simulink model "realTimeBatteryOPC"  (R2024a)
settings: Solver=FixedStepAuto  StartTime=0.0  StopTime=150000  RelTol=1e-3
values from neighbouring files (symbols this model uses):
  A = 0.00110214    [ConfiguracaoInicial.m]
  B = 0.000233175'    [ConfiguracaoInicial.m]
  C = 7.6408e-8    (= 7.6408e-08)    [ConfiguracaoInicial.m]
  cutoffVoltage = 3.65    [ConfiguracaoInicial.m]
  dischargeCutoffVoltage = 1.8    [ConfiguracaoInicial.m]
  finalPulse = 14    [ConfiguracaoInicial.m]
  hppcPulses = [0.05,0.05,0.05,0.05,0.1,0.1,0.1,0.1,0.1,0.1,0.05,0.05,0.05,0.05]    [ConfiguracaoInicial.m]
  initialCapacity = 1.45383    [ConfiguracaoInicial.m]
  initialSOC = 1.0    (= 1)    [ConfiguracaoInicial.m]
  initialState = 11    [ConfiguracaoInicial.m]
  loadCurrent = 1.45383    [ConfiguracaoInicial.m]
  maxCurrent = 100000000000000    [ConfiguracaoInicial.m]
  maxSOC = 10000000000.5    [ConfiguracaoInicial.m]
  maxTemperature = 800000000    [ConfiguracaoInicial.m]
  maxVoltage = 10000000.0    (= 10000000)    [ConfiguracaoInicial.m]
  minCurrent = -1000000000000    [ConfiguracaoInicial.m]
  minSOC = -10000000000.5    [ConfiguracaoInicial.m]
  minTemperature = -1500000    [ConfiguracaoInicial.m]
  minVoltage = -100000    [ConfiguracaoInicial.m]
  restChargeTimeHPPC = 3600*3    (= 10800)    [ConfiguracaoInicial.m]
  restTimeHPPC = 3600*2    (= 7200)    [ConfiguracaoInicial.m]
  Rt = 10000    [ConfiguracaoInicial.m]
  sampleTime = 0.01    [ConfiguracaoInicial.m]
  startDelay = 100    [ConfiguracaoInicial.m]
  startPulse = 1    [ConfiguracaoInicial.m]
undefined symbols (not defined in the file or in its folder): National_Instruments, PCIe, Standard_Devices, TCP_Protocol
libraries: eeGeneralControl x6, sldrtlib x5, slpidlib x1
settings Model: SimulationMode=external  ExtModeTrigDuration=180000  ExtModeArchiveMode=auto  ExtModeArchiveFileName=TesteComunicacao  ExtModeArchiveDirName=C:\Users\proje\OneDrive\Área de Trabalho\RealTimeBattery\Resultados Comunicacao  ExtModeWriteAllDataToWs=on  Creator=User  LastModifiedBy=proje
settings SolverCC: AlgebraicLoopSolver=TrustRegion  AutoInsertRateTranBlk=on  DecoupledContinuousIntegration=on  MinimalZcImpactIntegration=on
settings DataIOCC: ReturnWorkspaceOutputs=off
settings DebuggingCC: UnconnectedInputMsg=warning  UnconnectedOutputMsg=warning  UnconnectedLineMsg=warning  ArithmeticOperatorsInVariantConditions=warning
settings HardwareCC: ProdBitPerLong=64  ProdHWDeviceType=Intel->x86-64 (Linux 64)
settings ModelReferenceCC: EnableRefExpFcnMdlSchedulingChecks=on
settings SFSimCC: SimUseLocalCustomCode=off  CustomCodeUndefinedFunction=UseInterfaceOnly
settings RTWCC: Description=Simulink Desktop Real-Time  SystemTargetFile=sldrt.tlc  TemplateMakefile=sldrt.tmf  RTWUseLocalCustomCode=off  RTWCompilerOptimization=on  GPUComputeCapability=3.5  DLArmComputeVersion=19.05
settings CodeAppCC: MaxIdLength=95
settings SimulinkDesktopRealTimeCC: TargetLibSuffix=_sldrt.a  TargetPreCompLibLocation=C:\Program Files\MATLAB\R2024a\toolbox\sldrt\lib\win64
settings ConfigsetCC: ListOpcUaClients=[]  EndPoints=[]

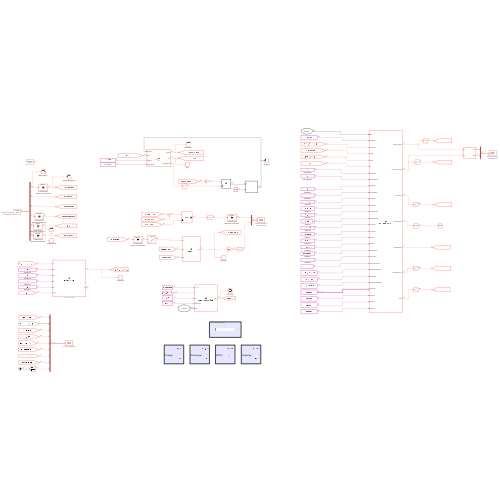
[thumbnail: Simulink's stored preview of the top-level diagram]
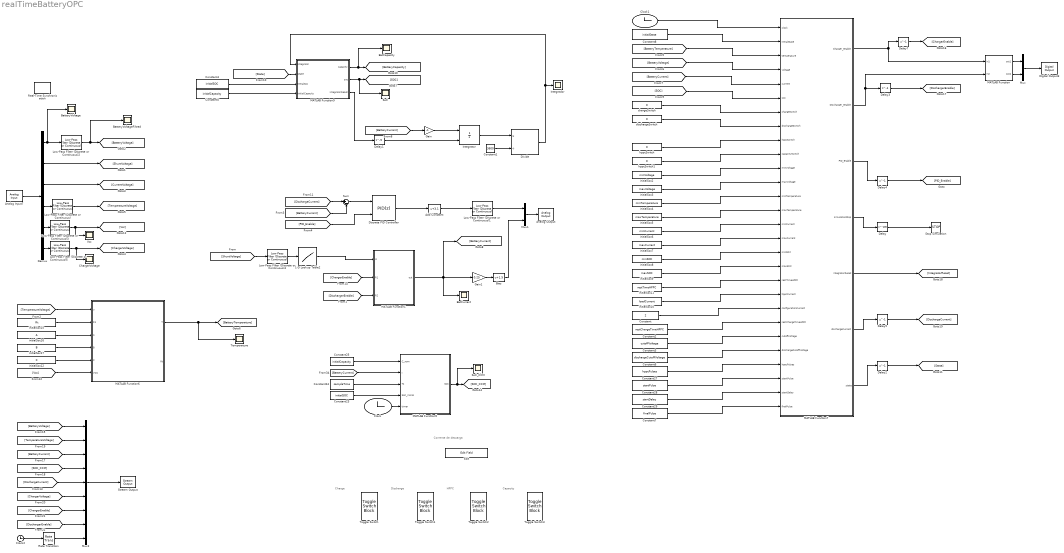
== system realTimeBatteryOPC ==
  note: Corrente de descarga
  note: Charge
  note: Discharge
  note: HPPC
  note: Capacity
  1-D Lookup Table2 : Lookup_n-D  NumberOfTableDimensions=1  BreakpointsForDimension1=|  Table=|  InternalRulePriority=Speed  RndMeth=Simplest
      BreakpointsForDimension1=|
      | [-0.703368941137097
      | -0.562690330092723
      | -0.492566163770883
      | -0.422967022263301
      | -0.352467845069619
      | -0.282288882664180
      | -0.247102233547827
      | -0.211796157294334
      | -0.176436693515434
      | -0.141402369117175
      | -0.106070485459359
      | -0.070887043775281
      | -0.035430249481695
      | -0.000072010558515
      | 0.035179496254845
      | 0.070319440336417
      | 0.105617401894233
      | 0.141115276831389
      | 0.176018947968660
      | 0.211326591943553
      | 0.246422461552550
      | 0.281747789595088
      | 0.351752022865883
      | 0.421762375644377
      | 0.491793233279879
      | 0.561360569786677
      | 0.701503863747804
      | ]
      Table=|
      | [-5.0040
      | -3.9980
      | -3.4995
      | -3.0010
      | -2.4995
      | -2.0000
      | -1.7500
      | -1.4990
      | -1.2490
      | -1.0005
      | -0.7495
      | -0.4995
      | -0.2490
      | 0.0000
      | 0.2500
      | 0.5000
      | 0.7500
      | 1.0020
      | 1.2505
      | 1.5005
      | 1.7505
      | 2.0020
      | 2.5000
      | 3.0000
      | 3.5005
      | 3.9985
      | 5.0025]
  Add Constant : Bias  Bias=3.1  SaturateOnIntegerOverflow=off
  Analog Input7 : sldrtlib/Analog Input  SampleTime=sampleTime  MaxMissedTicks=missedTicks  ShowMissedTicks=off  YieldWhenWaiting=off  DrvName=National_Instruments/PCIe-6323  DrvAddress=4294967295  DrvOptions=[1 127 63 0 0 0 0]  Channels=[1,2,3,4,5,6]  RangeMode=1  VoltRange=1  DataType=1
      settings: AttributesFormatString=National Instruments\nPCIe-6323 [auto]
  Analog Output : sldrtlib/Analog Output  SampleTime=sampleTime  MaxMissedTicks=missedTicks  ShowMissedTicks=off  YieldWhenWaiting=off  DrvName=National_Instruments/PCIe-6323  DrvAddress=4294967295  DrvOptions=[1 127 63 0 0 0 0]  Channels=[1,2]  RangeMode=1  VoltRange=1  InitialValue=0  FinalValue=0
      settings: AttributesFormatString=National Instruments\nPCIe-6323 [auto]
  BatCapacity : Scope
  BatCurrent : Scope
  BatteryVoltage : Scope
  BatteryVoltageFiltred : Scope
  Bias : Bias  Bias=1.5  SaturateOnIntegerOverflow=off
  ChargerVoltage : Scope
  Clock : Clock
  Clock1 : Clock
  Clock2 : Clock
  Constant : Constant  Value=2
  Constant1 : Constant  Value=3600
  Constant2 : Constant  Value=restChargeTimeHPPC
  Constant23 : Constant  Value=initialSOC
  Constant24 : Constant  Value=sampleTime
  Constant25 : Constant  Value=initialCapacity
  Constant27 : Constant  Value=hppcPulses
  Constant28 : Constant  Value=startPulse
  Constant29 : Constant  Value=startDelay
  Constant3 : Constant  Value=cutoffVoltage
  Constant4 : Constant  Value=initialSOC
  Constant5 : Constant  Value=initialCapacity
  Constant6 : Constant  Value=dischargeCutoffVoltage
  Constant7 : Constant  Value=finalPulse
  Constant8 : Constant  Value=initialState
  Delay : Delay  DelayLength=100  InitialCondition=0  SampleTime=sampleTime
  Delay1 : Delay  DelayLength=5  InitialCondition=0  SampleTime=sampleTime
  Delay2 : Delay  DelayLength=1  InitialCondition=0  SampleTime=sampleTime
  Delay{3..5,7} (4 alike) : Delay  DelayLength=1  InitialCondition=1  SampleTime=sampleTime
  Demux : Demux  Outputs=6
  Digital Output3 : sldrtlib/Digital Output  SampleTime=sampleTime  MaxMissedTicks=missedTicks  ShowMissedTicks=off  YieldWhenWaiting=off  DrvName=National_Instruments/PCIe-6323  DrvAddress=4294967295  DrvOptions=[1 127 63 0 0 0 0]  Channels=[2,1]  BitMode=1  InitialValue=[]  FinalValue=[]
      settings: AttributesFormatString=National Instruments\nPCIe-6323 [auto]
  Discrete PID Controller : slpidlib/PID Controller  Controller=PID  Form=Ideal  TimeDomain=Discrete-time  UseExternalTs=off  SampleTime=sampleTime  IntegratorMethod=Forward Euler  FilterMethod=Forward Euler  ControllerParametersSource=internal  P=0.07  I=0.007  UseKiTs=on  D=0.7  UseExternalDerivativeSource=off  N=10  UseFilter=on  TunerSelectOption=Transfer Function Based (PID Tuner App)  ZeroCross=off  InitialConditionSource=internal  InitialConditionForIntegrator=0  InitialConditionForFilter=0  DifferentiatorICPrevScaledInput=0  ExternalReset=level  TrackingMode=off  Kt=1  LimitOutput=on  SatLimitsSource=internal  UpperSaturationLimit=7  LowerSaturationLimit=0  LinearizeAsGain=off  AntiWindupMode=clamping  Kb=1  LimitIntegrator=off  UpperIntegratorSaturationLimit=5  LowerIntegratorSaturationLimit=-5  POutMin=[]  POutMax=[]  IOutMin=[]  IOutMax=[]  DOutMin=[]  DOutMax=[]  NOutMin=[]  NOutMax=[]  SumOutMin=[]  SumOutMax=[]  SaturationOutMin=[]  SaturationOutMax=[]  PParamMin=[]  PParamMax=[]  IParamMin=[]  IParamMax=[]  DParamMin=[]  DParamMax=[]  NParamMin=[]  NParamMax=[]  KbParamMin=[]  KbParamMax=[]  KtParamMin=[]  KtParamMax=[]  KbOutMin=[]  KbOutMax=[]  KtOutMin=[]  KtOutMax=[]  IntegratorOutMin=[]  IntegratorOutMax=[]  FilterOutMin=[]  FilterOutMax=[]  SumI1OutMin=[]  SumI1OutMax=[]  SumI2OutMin=[]  SumI2OutMax=[]  SumI3OutMin=[]  SumI3OutMax=[]  SumI4OutMin=[]  SumI4OutMax=[]  SumDOutMin=[]  SumDOutMax=[]  DifferentiatorOutMin=[]  DifferentiatorOutMax=[]  FilterDiffOutCoefMin=[]  FilterDiffOutCoefMax=[]  ReciprocalOutMin=[]  ReciprocalOutMax=[]  SumDenOutMin=[]  SumDenOutMax=[]  SumNumOutMin=[]  SumNumOutMax=[]  DivideOutMin=[]  DivideOutMax=[]  UdiffTsProdOutMin=[]  UdiffTsProdOutMax=[]  NTsProdOutMin=[]  NTsProdOutMax=[]  UintegralTsProdOutMin=[]  UintegralTsProdOutMax=[]  UngainTsProdOutMin=[]  UngainTsProdOutMax=[]  ClampingZeroOutDataTypeStr=Inherit: Inherit via back propagation  ClampingZeroOutMin=[]  ClampingZeroOutMax=[]  FilterDenConstantOutDataTypeStr=Inherit: Inherit via back propagation  FilterDenConstantOutMin=[]  FilterDenConstantOutMax=[]  PCopyOutDataTypeStr=Inherit: Inherit via back propagation  PCopyOutMin=[]  PCopyOutMax=[]  NCopyOutDataTypeStr=Inherit: Inherit via back propagation  NCopyOutMin=[]  NCopyOutMax=[]  IntegratorContinuousStateAttributes=''  IntegratorStateMustResolveToSignalObject=off  IntegratorRTWStateStorageClass=Auto  FilterContinuousStateAttributes=''  FilterStateMustResolveToSignalObject=off  FilterRTWStateStorageClass=Auto  ParallelPVariant=Passthrough  IdealPVariant=InternalParameters  IVariant=InternalParameters  DVariant=InternalParameters  IntegratorVariant=Discrete  SatVariant=Enabled  AWVariant=DiscClampingIdeal  PCopyVariant=InternalParamsIdeal  TRVariant=Disabled  FdbkBlocksVariant=Forward  IdealPFdbkVariant=Disabled  SatFdbkVariant=Disabled  DerivativeFilterVariant=ForwardEulerFilter  NVariant=InternalParameters  NCopyVariant=Disabled  FilterICVariant=InternalICsFilter  IntegratorICVariant=InternalICs  ExternalResetVariant=ExternalReset  TRSumVariant=Passthrough  SumFdbkVariant=Disabled  SumVariant=Sum_PID  TsampFilterVariant=InternalTs  TsampNgainVariant=Passthrough  TsampIntegralVariant=Disabled_SignalSpec  ExternalSaturationOutDataTypeStr=Inherit: Same as second input  DerivativeSourceVariant=ErrorSignal
      settings: LibrarySourceBlock=simulink/Discrete/Discrete PID Controller
  Divide : Product  Inputs=*/
  Edit : EditField  LabelPosition=Hide  ShowInitialText=on  Alignment=Center
  Gain : Gain  Gain=-1
  Gain1 : Gain  Gain=0.25
  Integrador : Scope
  Integrator : Integrator  ExternalReset=rising
  Low-Pass Filter (Discrete or Continuous) : eeGeneralControl/Low-Pass Filter (Discrete or Continuous)  K=1  T=1  B=inf  A=-inf  init_option=Specify as parameter  x0=2.5  Ts=sampleTime
  Low-Pass Filter (Discrete or Continuous)1 : eeGeneralControl/Low-Pass Filter (Discrete or Continuous)  K=1  T=1  B=inf  A=-inf  init_option=Specify as parameter  x0=0  Ts=sampleTime
  Low-Pass Filter (Discrete or Continuous)2 : eeGeneralControl/Low-Pass Filter (Discrete or Continuous)  K=1  T=1  B=inf  A=-inf  init_option=Specify as parameter  x0=0  Ts=sampleTime
  Low-Pass Filter (Discrete or Continuous)3 : eeGeneralControl/Low-Pass Filter (Discrete or Continuous)  K=1  T=1  B=inf  A=-inf  init_option=Specify as parameter  x0=5  Ts=sampleTime
  Low-Pass Filter (Discrete or Continuous)4 : eeGeneralControl/Low-Pass Filter (Discrete or Continuous)  K=1  T=1  B=inf  A=-inf  init_option=Specify as parameter  x0=0  Ts=sampleTime
  Low-Pass Filter (Discrete or Continuous)5 : eeGeneralControl/Low-Pass Filter (Discrete or Continuous)  K=1  T=1  B=inf  A=-inf  init_option=Specify as parameter  x0=3  Ts=sampleTime
  MATLAB Function : MATLAB Function  TreatAsAtomicUnit=on  SystemSampleTime=sampleTime
  MATLAB Function1 : MATLAB Function  TreatAsAtomicUnit=on  SystemSampleTime=sampleTime
  MATLAB Function5 : MATLAB Function  TreatAsAtomicUnit=on  SystemSampleTime=sampleTime
  MATLAB Function6 : MATLAB Function  TreatAsAtomicUnit=on  SystemSampleTime=sampleTime
  MATLAB Function7 : MATLAB Function  TreatAsAtomicUnit=on  SystemSampleTime=sampleTime
  MATLAB Function9 : MATLAB Function  TreatAsAtomicUnit=on  SystemSampleTime=sampleTime
  Mux : Mux  Inputs=2
  Mux1 : Mux  Inputs=2
  Mux2 : Mux  Inputs=9
  Rate Transition : RateTransition  OutPortSampleTime=sampleTime
  Real-Time Synchronization : sldrtlib/Real-Time Synchronization  SampleTime=sampleTime  MaxMissedTicks=missedTicks  ShowMissedTicks=on  YieldWhenWaiting=off
  SoC : Scope
  SoC_CCM : Scope
  Stop Simulation : Stop
  Stream Output : sldrtlib/Stream Output  SampleTime=sampleTime  MaxMissedTicks=10  ShowMissedTicks=off  YieldWhenWaiting=off  DrvName=Standard_Devices/TCP_Protocol  DrvAddress=16384  DrvOptions=[0 8081 49 57 50 46 49 54 56 46 48 46 50 51 49 0 0 0 0 0 0 0 0 0 0 0 0 0 0 0 0 0 0 0 0 0 0 0 0 0 0 0 0 0 0 0 0 0 0 0 0 0 0 0 0 0 0 0 0 0 0 0 0 0 0 0 0 0 0 0 0 0 0 0 0 0 0 0 0 0 0 0 0 0 0 0 0 0 0 0 0 0 0 0 0 0 0 0 0 0 0 0 0 0 0 0 0 0 0 0 0 0 0 0 0 0 0 0 0 0 0 0 0 0 0 0 0 0 0 0 0 0 0 0 0 0 0 0 0 0 0 0 0 0 0 0 0 0 0 0 0 0 0 0 0 0 0 0 0 0 0 0 0 0 0 0 0 0 0 0 0 0 0 0 0 0 0 0 0 0 0 0 0 0 0 0 0 0 0 0 0 0 0 0 0 0 0 0 0 0 0 0 0 0 0 0 0 0 0 0 0 0 0 0 0 0 0 0 0 0 0 0 0 0 0 0 0 0 0 0 0 0 0 0 0 0 0 0 0 0 0 0 0 0 0 0 0 0 0 0 0 0 0 0 0 0]  PortSizes=9  FormatString="\"<%lf:%lf:%lf:%lf:%lf:%lf:%lf:%lf:%lf>\""  ShowReady=off  ShowError=off  InitialValue=[]  FinalValue=[]
      settings: AttributesFormatString=TCP Protocol [16384]
  Sum : Sum  Inputs=|+-
  Temperature : Scope
  Toggle Switch{,1..3} (4 alike) : ToggleSwitchBlock
      settings: Values={{'Off', 'On'}, [0 1]}
  Vcc : Scope
  chargeSwitch : Constant  Value=0
  dischargeSwitch : Constant  Value=0
  hppcSwitch : Constant  Value=0
  hppcSwitch1 : Constant  Value=0
  initialSoc10 : Constant  Value=loadCurrent
  initialSoc11 : Constant  Value=restTimeHPPC
  initialSoc12 : Constant  Value=C
  initialSoc15 : Constant  Value=Rt
  initialSoc16 : Constant  Value=A
  initialSoc17 : Constant  Value=B
  initialSoc2 : Constant  Value=minVoltage
  initialSoc3 : Constant  Value=maxVoltage
  initialSoc4 : Constant  Value=minTemperature
  initialSoc5 : Constant  Value=maxTemperature
  initialSoc6 : Constant  Value=minCurrent
  initialSoc7 : Constant  Value=maxCurrent
  initialSoc8 : Constant  Value=minSOC
  initialSoc9 : Constant  Value=maxSOC
  wires:
  Clock1/1 -> MATLAB Function7/1(clock)
  MATLAB Function7/1(Charger_Enable) -> Delay7/1, MATLAB Function/1(in1)
  Demux/1 -> Low-Pass Filter (Discrete or Continuous)2/1, BatteryVoltage/1
  [BatteryTemperature] -> MATLAB Function7/3(temperature)
  [BatteryVoltage] -> MATLAB Function7/4(voltage)
  [BatteryCurrent] -> MATLAB Function7/5(current)
  Gain/1 -> Integrator/1
  [BatteryCurrent] -> Gain/1
  [SOC] -> MATLAB Function7/6(soc)
  MATLAB Function7/4(simulationStop) -> Delay/1
  Delay/1 -> Stop Simulation/1
  initialSoc4/1 -> MATLAB Function7/13(minTemperature)
  initialSoc3/1 -> MATLAB Function7/12(maxVoltage)
  initialSoc2/1 -> MATLAB Function7/11(minVoltage)
  initialSoc5/1 -> MATLAB Function7/14(maxTemperature)
  initialSoc6/1 -> MATLAB Function7/15(minCurrent)
  initialSoc7/1 -> MATLAB Function7/16(maxCurrent)
  initialSoc8/1 -> MATLAB Function7/17(minSOC)
  initialSoc9/1 -> MATLAB Function7/18(maxSOC)
  initialSoc11/1 -> MATLAB Function7/19(restTimeHPPC)
  initialSoc15/1 -> MATLAB Function6/2(R1)
  chargeSwitch/1 -> MATLAB Function7/7(chargeSwitch)
  dischargeSwitch/1 -> MATLAB Function7/8(dischargeSwitch)
  hppcSwitch/1 -> MATLAB Function7/9(hppcSwitch)
  [BatteryCurrent] -> Sum/2
  Sum/1 -> Discrete PID Controller/1
  Integrator/1 -> Divide/1
  Constant1/1 -> Divide/2
  initialSoc10/1 -> MATLAB Function7/20(hppcCurrent)
  MATLAB Function7/5(integratorReset) -> [IntegratorReset]
  MATLAB Function7/6(dischargeCurrent) -> Delay5/1
  [DischargeCurrent] -> Sum/1
  MATLAB Function9/1(capacity) -> BatCapacity/1, [BatteryCapacity]
  MATLAB Function9/2(soc) -> SoC/1, [SOC]
  Delay1/1 -> Integrator/2
  [State] -> MATLAB Function9/2(state)
  [TemperatureVoltage] -> MATLAB Function6/1(u)
  initialSoc12/1 -> MATLAB Function6/5(C)
  initialSoc17/1 -> MATLAB Function6/4(B)
  initialSoc16/1 -> MATLAB Function6/3(A)
  Constant/1 -> MATLAB Function7/21(configurationCurrent)
  Constant2/1 -> MATLAB Function7/22(restChargeTimeHPPC)
  Delay3/1 -> [DischargerEnable]
  MATLAB Function7/2(Discharger_Enable) -> MATLAB Function/2(in2), Delay3/1
  MATLAB Function7/3(PID_Enable) -> Delay4/1
  Delay4/1 -> [PID_Enable]
  Delay5/1 -> [DischargeCurrent]
  MATLAB Function7/7(state) -> Delay2/1
  MATLAB Function9/3(integratorReset) -> Delay1/1
  Constant3/1 -> MATLAB Function7/23(cutoffVoltage)
  Constant4/1 -> MATLAB Function9/3(initialSoc)
  Constant5/1 -> MATLAB Function9/4(initialCapacity)
  Delay2/1 -> [State]
  Divide/1 -> MATLAB Function9/1(integrator), Integrador/1
  Constant8/1 -> MATLAB Function7/2(initialState)
  [Vcc] -> MATLAB Function6/6(VCC)
  hppcSwitch1/1 -> MATLAB Function7/10(capacitySwitch)
  [ShuntVoltage] -> Low-Pass Filter (Discrete or Continuous)4/1
  Low-Pass Filter (Discrete or Continuous)4/1 -> 1-D Lookup Table2/1
  Gain1/1 -> Bias/1
  Constant24/1 -> MATLAB Function5/3(Ts)
  [BatteryCurrent] -> MATLAB Function5/2(I)
  MATLAB Function5/1(SoC) -> SoC_CCM/1, [SOC_CCM]
  Constant25/1 -> MATLAB Function5/1(C_nom)
  Clock/1 -> MATLAB Function5/5(timer)
  Analog Input7/1 -> Demux/1
  Mux/1 -> Digital Output3/1
  Constant27/1 -> MATLAB Function7/25(hppcPulses)
  Constant28/1 -> MATLAB Function7/26(startPulse)
  Constant29/1 -> MATLAB Function7/27(startDelay)
  Constant23/1 -> MATLAB Function5/4(SoC_Inicial)
  Bias/1 -> Mux1/2
  Mux1/1 -> Analog Output/1
  Demux/6 -> Low-Pass Filter (Discrete or Continuous)5/1
  Demux/5 -> Low-Pass Filter (Discrete or Continuous)3/1
  Demux/4 -> Low-Pass Filter (Discrete or Continuous)/1
  Demux/2 -> [ShuntVoltage]
  Demux/3 -> [CurrentVoltage]
  [PID_Enable] -> Discrete PID Controller/2
  Discrete PID Controller/1 -> Add Constant/1
  Add Constant/1 -> Low-Pass Filter (Discrete or Continuous)1/1
  Low-Pass Filter (Discrete or Continuous)1/1 -> Mux1/1
  Constant6/1 -> MATLAB Function7/24(dischargeCutoffVoltage)
  Constant7/1 -> MATLAB Function7/28(finalPulse)
  1-D Lookup Table2/1 -> MATLAB Function1/1(in)
  [ChargerEnable] -> MATLAB Function1/2(R1)
  [DischargerEnable] -> MATLAB Function1/3(R2)
  MATLAB Function1/1(out) -> [BatteryCurrent], BatCurrent/1, Gain1/1
  Low-Pass Filter (Discrete or Continuous)2/1 -> BatteryVoltageFiltred/1, [BatteryVoltage]
  Delay7/1 -> [ChargerEnable]
  [BatteryVoltage] -> Mux2/1
  Mux2/1 -> Stream Output/1
  [TemperatureVoltage] -> Mux2/2
  [BatteryCurrent] -> Mux2/3
  [SOC_CCM] -> Mux2/4
  [ChargerVoltage] -> Mux2/6
  [ChargerEnable] -> Mux2/7
  [DischargerEnable] -> Mux2/8
  Clock2/1 -> Rate Transition/1
  Rate Transition/1 -> Mux2/9
  [DischargeCurrent] -> Mux2/5
  MATLAB Function/2(out2) -> Mux/2
  MATLAB Function/1(out1) -> Mux/1
  MATLAB Function6/1(T) -> Temperature/1, [BatteryTemperature]
  Low-Pass Filter (Discrete or Continuous)/1 -> [TemperatureVoltage]
  Low-Pass Filter (Discrete or Continuous)3/1 -> Vcc/1, [Vcc]
  Low-Pass Filter (Discrete or Continuous)5/1 -> ChargerVoltage/1, [ChargerVoltage]

== matlab function realTimeBatteryOPC/MATLAB Function9 ==
  data: integrator input; state input; capacity output; soc output; integratorReset output; initialSoc input; initialCapacity input
function [capacity, soc, integratorReset] = calculate_capacity(integrator, state, initialSoc,initialCapacity)
    persistent current_capacity; % Definindo a capacidade como persistente
    persistent socRef;
    persistent previousState;
    
    if isempty(current_capacity) % Verificando se a capacidade atual está vazia
        current_capacity = initialCapacity; % Definindo a capacidade inicial como zero
        socRef=initialSoc;
        previousState=0;
    end
    integratorReset=0;

    if state==1 && previousState==0
        socRef=0;
        integratorReset=1;
    elseif state==4 && previousState==3 && abs(integrator)> current_capacity
        current_capacity = abs(integrator); 
        integratorReset=1;
        socRef=1;
    elseif state==5 && previousState==4
        integratorReset=1;
        socRef=1;
    elseif state==6 && previousState==5 && abs(integrator)>current_capacity
        current_capacity = abs(integrator); 
        integratorReset=1;
        socRef=0;
    elseif state==7 && previousState==6
        integratorReset=1;
        socRef=0;
    elseif state==10 && previousState==9 && abs(integrator)>current_capacity
        %current_capacity = abs(integrator); 
        integratorReset=1;
        socRef=1;
    elseif state==11 && previousState==1-0 
        integratorReset=1;
        socRef=1;
    end
    
    previousState=state;

    capacity = current_capacity; % Retornando a capacidade atual

    soc=socRef+integrator/current_capacity;

    if(soc<-0.1) 
        soc=-0.1;
    end

    if(soc>1.1) 
        soc=1.1;
    end
end

== matlab function realTimeBatteryOPC/MATLAB Function1 ==
  data: in input; R1 input; R2 input; out output
function out  = currentOn(in, R1, R2) 

    if(R1==1 || R2==1)
        out=in;
    else
        out=0;
    end

end

== matlab function realTimeBatteryOPC/MATLAB Function ==
  data: in1 input; out1 output; in2 input; out2 output
function [out1, out2] = fcn(in1, in2)
    % Definir variáveis persistentes para armazenar o estado anterior
    persistent previousIn2;
    
    % Inicializar as variáveis persistentes na primeira execução
    if isempty(previousIn2)
        previousIn2 = 0;
    end

    if(previousIn2==0 && in2==1)
        out1=0;
        out2=1;
    elseif(previousIn2==1 && in2==0)
        out1=0;
        out2=1;
    elseif(in2==1)
        out2=1;
        out1=1;
    else
        out2=0;
        out1=in1;
    end

    
    previousIn2=in2;

end

== matlab function realTimeBatteryOPC/MATLAB Function5 ==
  data: C_nom input; SoC output; I input; Ts input; SoC_Inicial input; timer input
function SoC = coulomb_counting_SOC(C_nom, I, Ts, SoC_Inicial,timer)
% Este código implementa a contagem de Coulomb usando um integrador discreto
% com o método do trapézio, utilizando variáveis persistentes.
% C_nom: Capacidade nominal da bateria (Ah)
% I: Corrente da bateria (A)
% Ts: Tempo de amostragem (s)

% Variáveis persistentes para armazenar o SoC e a corrente anterior
persistent SoC_prev I_prev;
if(timer>100)
    if isempty(SoC_prev)
        SoC_prev = SoC_Inicial; % Estado de carga inicial, ajuste conforme necessário
    end
    if isempty(I_prev)
        I_prev = 0;
    end
    
    % Integração pelo método do trapézio
    dSoC = 0.99* (I + I_prev) * Ts / (2 * C_nom * 3600);
    
    % Atualizar o estado de carga
    SoC = SoC_prev - dSoC;
    
    % Garantir que o SoC esteja dentro dos limites [0, 100]%
    SoC = max(min(SoC, 1), 0);
    
    % Atualizar as variáveis persistentes
    SoC_prev = SoC;
    I_prev = I;
        
else
    SoC=1;
end
end

== matlab function realTimeBatteryOPC/MATLAB Function6 ==
  data: u input; R1 input; A input; T output; Rt output; B input; C input; VCC input
function [T, Rt] = temperatureCalc(u, R1, A, B, C, VCC) 

    if(u-R1~=0)
        Rt=(VCC*R1)/u - R1;
    else
        Rt=10000.
    end
    if((A+B*log(Rt)+C*(log(Rt))^3)~=0)
        T=1/(A+B*log(Rt)+C*(log(Rt))^3);
    else
        T=293.15;
    end
    T=T-273.15;

end

== matlab function realTimeBatteryOPC/MATLAB Function7 ==
  data: clock input; initialState input; Charger_Enable output; temperature input; voltage input; current input; soc input; chargeSwitch input; dischargeSwitch input; hppcSwitch input; capacitySwitch input; minVoltage input; maxVoltage input; minTemperature input; maxTemperature input; minCurrent input; maxCurrent input; minSOC input; maxSOC input; restTimeHPPC input; hppcCurrent input; configurationCurrent input; Discharger_Enable output; PID_Enable output; simulationStop output; integratorReset output; dischargeCurrent output; restChargeTimeHPPC input; state output; cutoffVoltage input; dischargeCutoffVoltage input; hppcPulses input; startPulse input; startDelay input; finalPulse input
function [Charger_Enable, Discharger_Enable, PID_Enable, simulationStop, integratorReset, dischargeCurrent,state] = MATLAB_Function7(clock, initialState, temperature, voltage, current, soc, ...
    chargeSwitch, dischargeSwitch, hppcSwitch, capacitySwitch, minVoltage, maxVoltage, minTemperature, maxTemperature, ...
    minCurrent, maxCurrent, minSOC, maxSOC, restTimeHPPC, hppcCurrent, configurationCurrent,restChargeTimeHPPC, cutoffVoltage,dischargeCutoffVoltage, hppcPulses, startPulse, startDelay,finalPulse)

persistent previousState;
persistent counter;
persistent HPPCState;
persistent lastSOC;
persistent dischargeCounter;
persistent stack;
persistent currentMean;
persistent previousSwitchHPPC;
persistent previousSwitchCharge;



persistent stackTop;
simulationStop=false;


if(isempty(previousState))
    previousState=0;
    previousSwitchCharge=0;
    previousSwitchHPPC=0;
    currentMean=0;
    counter=clock;
    HPPCState=0;
    dischargeCounter=startPulse;
    lastSOC=1;
    stack=hppcPulses;
    stackTop=0.1;
end

integratorReset=0;


if(chargeSwitch~=previousSwitchCharge && chargeSwitch==1)
    counter=clock;
else
    if(hppcSwitch~=previousSwitchHPPC && hppcSwitch==1)
        counter=clock;
    end
end
dischargeCurrent=configurationCurrent;
if(temperature>maxTemperature || temperature<minTemperature || voltage>maxVoltage || voltage<minVoltage || current>maxCurrent || current<minCurrent || soc>maxSOC || soc<minSOC)
    Charger_Enable=1;
    Discharger_Enable=1;
    PID_Enable=1;
    simulationStop=true;
else
    if chargeSwitch
        Charger_Enable=1;
        Discharger_Enable=0;
        PID_Enable=1;

    else
        if dischargeSwitch
            Charger_Enable=0;
            Discharger_Enable=1;
            PID_Enable=0;
        else
            if hppcSwitch || capacitySwitch
                dischargeCurrent=hppcCurrent;
                if(HPPCState==0)
                    Charger_Enable=0;
                    Discharger_Enable=0;
                    PID_Enable=1;
                    if(clock-counter>=startDelay)
                        counter=clock;
                        if(hppcSwitch)
                            HPPCState=initialState;
                        else
                            HPPCState=1;
                        end
                    end
                elseif(HPPCState==1)
                    Charger_Enable=1;
                    Discharger_Enable=0;
                    PID_Enable=1;
                    if(clock-counter>100 && current>-0.1)
                        currentMean=0;
                        counter=clock;
                        HPPCState=2;
                    end
                elseif(HPPCState==2)
                    Charger_Enable=1;
                    Discharger_Enable=0;
                    PID_Enable=1;

                    if(clock-counter>=50)
                        if(currentMean/50>-0.1)
                            counter=clock;
                            HPPCState=3;
                        else
                            counter=clock;
                            HPPCState=1;
                        end
                    end
                elseif(HPPCState==3)
                    Charger_Enable=0;
                    Discharger_Enable=0;
                    PID_Enable=1;
                    if(clock-counter>restChargeTimeHPPC)
                        integratorReset=1;
                        counter=clock;
                        HPPCState=4;
                    end
                elseif(HPPCState==4)
                    Charger_Enable=0;
                    Discharger_Enable=1;
                    PID_Enable=0;
                    if(clock-counter>100 && voltage<dischargeCutoffVoltage)
                        counter=clock;
                        HPPCState=5;
                        integratorReset=1;
                    end
                elseif(HPPCState==5)
                    Charger_Enable=0;
                    Discharger_Enable=0;
                    PID_Enable=1;
                    if(clock-counter>restTimeHPPC)
                        counter=clock;
                        HPPCState=6;
                        integratorReset=1;
                    end
                elseif(HPPCState==6)
                    Charger_Enable=1;
                    Discharger_Enable=0;
                    PID_Enable=1;
                    if(clock-counter>100 && current>-0.1)
                        counter=clock;
                        HPPCState=7;
                    end
                elseif(HPPCState==7)
                    Charger_Enable=1;
                    Discharger_Enable=0;
                    PID_Enable=1;
                    if(clock-counter>=50)
                        if(currentMean/50>-0.1)
                            counter=clock;
                            HPPCState=8;
                            integratorReset=1;
                        else
                            counter=clock;
                            HPPCState=6;
                        end
                    end
                elseif(HPPCState==8)
                    Charger_Enable=0;
                    Discharger_Enable=0;
                    PID_Enable=1;
                    if(clock-counter>restChargeTimeHPPC)
                        if(capacitySwitch)
                            simulationStop=true;
                        else
                            HPPCState=9;
                        end
                    end
                elseif(HPPCState==9)
                    Charger_Enable=0;
                    Discharger_Enable=0;
                    PID_Enable=1;
                    if(clock-counter>restChargeTimeHPPC)
                        counter=clock;
                        HPPCState=10;
                        lastSOC=soc;
                        stackTop=stack(dischargeCounter);
                    end
                elseif(HPPCState==10)
                    Charger_Enable=0;
                    Discharger_Enable=1;
                    PID_Enable=0;
                    if(lastSOC-soc>=stack(dischargeCounter))
                        dischargeCounter=dischargeCounter+1;
                        counter=clock;
                        HPPCState=11;
                    end
                elseif(HPPCState==11)
                    Charger_Enable=0;
                    Discharger_Enable=0;
                    PID_Enable=1;
                    if(clock-counter>=restTimeHPPC)
                        if(dischargeCounter>finalPulse || voltage<dischargeCutoffVoltage)
                            counter=clock;
                            HPPCState=12;
                        else
                            counter=clock;
                            HPPCState=10;
                            lastSOC=soc;
                            stackTop=stack(dischargeCounter);
                        end
                    end
                else
                    Charger_Enable=0;
                    Discharger_Enable=0;
                    PID_Enable=1;
                    if(clock-counter>restTimeHPPC*2)
                            simulationStop=true;
                    end
                end

            else
                Charger_Enable=0;
                Discharger_Enable=0;
                PID_Enable=1;
            end
        end
    end
end
previousSwitchHPPC=hppcSwitch;
previousSwitchCharge=chargeSwitch;
state=HPPCState;
end
